simulink model "TwoLinkManipulator_P_I_D"  (R2025a)
settings: Solver=VariableStepAuto  StartTime=0.0  StopTime=10.0  RelTol=1e-3
settings Model: Creator=jaisr  LastModifiedBy=jaisr

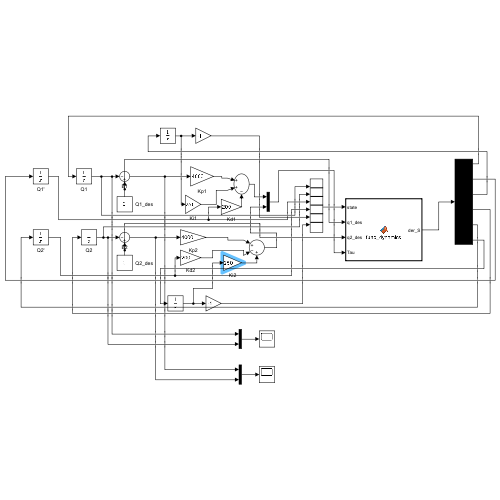
[thumbnail: Simulink's stored preview of the top-level diagram]
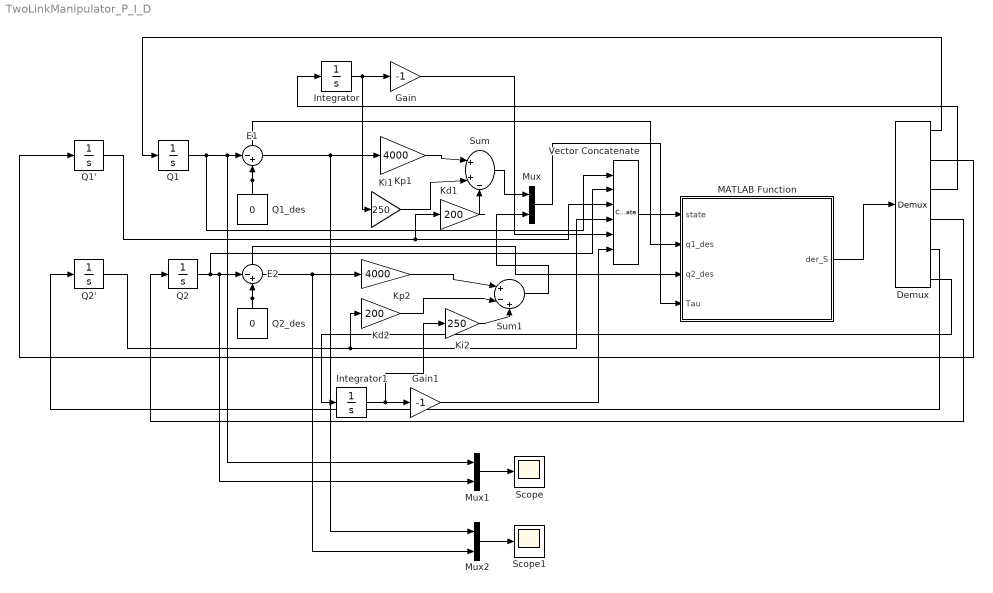
== system TwoLinkManipulator_P_I_D ==
  Demux : Demux  Outputs=6
  E1 : Sum  Inputs=|-+
  E2 : Sum  Inputs=|-+
  Gain : Gain  Gain=-1
  Gain1 : Gain  Gain=-1
  Integrator : Integrator
  Integrator1 : Integrator
  Kd1 : Gain  Gain=200
  Kd2 : Gain  Gain=200
  Ki1 : Gain  Gain=250
  Ki2 : Gain  Gain=250
  Kp1 : Gain  Gain=4000
  Kp2 : Gain  Gain=4000
  MATLAB Function : MATLAB Function  TreatAsAtomicUnit=on
  Mux : Mux  Inputs=2
  Mux1 : Mux  Inputs=2
  Mux2 : Mux  Inputs=2
  Q1 : Integrator  InitialCondition=0.2
  Q1' : Integrator
  Q1_des : Constant  Value=0
  Q2 : Integrator  InitialCondition=0.15
  Q2' : Integrator
  Q2_des : Constant  Value=0
  Scope : Scope
      settings: ActiveDisplayYMinimum=-0.8748046410340784  ActiveDisplayYMaximum=2.55962008935655
  Scope1 : Scope
      settings: ActiveDisplayYMinimum=-2.55962008935655  ActiveDisplayYMaximum=0.8748046410340784
  Sum : Sum  Inputs=|++-
  Sum1 : Sum  Inputs=|+-+
  Vector Concatenate : Concatenate  NumInputs=6
  wires:
  Mux1/1 -> Scope/1
  MATLAB Function/1(der_S) -> Demux/1
  Demux/4 -> Q2/1
  E1/1 -> Mux2/1, Kp1/1
  Demux/3 -> Integrator/1
  Kp2/1 -> Sum1/1
  Gain1/1 -> Vector Concatenate/6
  Vector Concatenate/1 -> MATLAB Function/1(state)
  Demux/2 -> Q1'/1
  Demux/5 -> Q2'/1
  Q1/1 -> Mux1/1, E1/1, Vector Concatenate/1
  Gain/1 -> Vector Concatenate/5
  Integrator/1 -> Ki1/1, Gain/1
  Mux/1 -> MATLAB Function/4(Tau)
  Q2_des/1 -> MATLAB Function/3(q2_des), E2/2
  Integrator1/1 -> Ki2/1, Gain1/1
  Mux2/1 -> Scope1/1
  Q2/1 -> Vector Concatenate/2, Mux1/2, E2/1
  Q1_des/1 -> MATLAB Function/2(q1_des), E1/2
  Q1'/1 -> Kd1/1, Vector Concatenate/3
  Demux/6 -> Integrator1/1
  Q2'/1 -> Kd2/1, Vector Concatenate/4
  Demux/1 -> Q1/1
  E2/1 -> Mux2/2, Kp2/1
  Kp1/1 -> Sum/1
  Kd1/1 -> Sum/3
  Ki1/1 -> Sum/2
  Sum/1 -> Mux/1
  Ki2/1 -> Sum1/3
  Kd2/1 -> Sum1/2
  Sum1/1 -> Mux/2

== matlab function TwoLinkManipulator_P_I_D/MATLAB Function ==
  data: state input; der_S output size=[6,1]; q1_des input; q2_des input; Tau input
function der_S = func_dynamics(state, q1_des, q2_des, Tau)
% This function represents the DYNAMICS ONLY, matching the project PDF.

    % System Parameters from Equation (8), (9), (10)
    m1 = 5;
    m2 = 3;
    l1 = 0.25;
    l2 = 0.15;
    g = 9.81;

    % Extracting state variables from the input 'state' vector
    q1 = state(1);
    q2 = state(2);
    q1dot = state(3);
    q2dot = state(4);
    % The integral error states are kept for PI/PID controller compatibility
    neg_int_q1 = state(5);
    neg_int_q2 = state(6);

    % Equations of motion from Equation (3) through (7)
    % M(q) — Inertia Matrix
    M11 = (m1 + m2)*l1^2 + m2*l2^2 + 2*m2*l1*l2*cos(q2);
    M12 = m2*l2*(l1*cos(q2) + l2);
    M21 = M12;
    M22 = m2*l2^2;
    M = [M11, M12; M21, M22];

    % C(q,q_dot) — Coriolis and Centrifugal Matrix
    c11 = -m2*l1*l2*sin(q2)*q2dot;
    c12 = -m2*l1*l2*sin(q2)*(q1dot + q2dot);
    c21 = 0; % As specified by the document's C matrix (Equation 6)
    c22 = m2*l1*l2*sin(q2)*q1dot;
    C = [c11, c12; c21, c22];

    % G(q) — Gravity Torque Vector
    g1 = m1*l1*g*cos(q1) + m2*g*(l2*cos(q1 + q2) + l1*cos(q1));
    g2 = m2*g*l2*cos(q1 + q2);
    G = [g1; g2];

    % Solve for q_ddot from M*q_ddot + C*q_dot + G = Tau
    q_ddot = M \ (Tau - C*[q1dot; q2dot] - G);

    % Calculate error for the integral state derivative
    q1_error = q1 - q1_des;
    q2_error = q2 - q2_des;

    % Return the state derivatives in the correct order
    der_S = [q1dot; q2dot; q_ddot(1); q_ddot(2); -q1_error; -q2_error];
end
